simulink library "ad_agg_scalar"  (R2017a)
settings: Solver=VariableStepAuto  StartTime=0.0  StopTime=10.0  RelTol=1e-3
libraries: autodiff x5
settings Model: Creator=eruffaldi  LastModifiedBy=eruffaldi

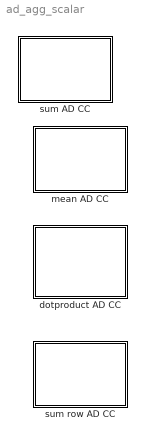
== system ad_agg_scalar ==
  dotproduct AD CC : Subsystem
  mean AD CC : Subsystem
  sum AD CC : Subsystem
  sum row AD CC : Subsystem
      mask Display: disp('Sum by ROW');

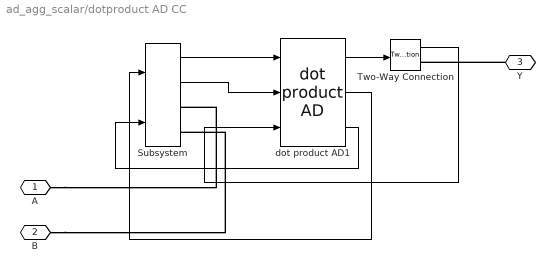
== system ad_agg_scalar/dotproduct AD CC ==
  Subsystem : autodiff/Plus AD CC/Subsystem
      settings: SourceProductName=AutoDiff
  Two-Way Connection : TwoWayConnection
  dot product AD1 : autodiff/dot product AD
      settings: SourceProductName=AutoDiff
  A : PMIOPort  Port=1  Side=Left
  B : PMIOPort  Port=2  Side=Left
  Y : PMIOPort  Port=3  Side=Right
  wires:
  dot product AD1/1 -> Two-Way Connection/1
  dot product AD1/3 -> Subsystem/2
  Subsystem/2 -> dot product AD1/2
  Two-Way Connection/1 -> dot product AD1/3
  dot product AD1/2 -> Subsystem/1
  Subsystem/1 -> dot product AD1/1
  connections:
  Y/RConn1 -- Two-Way Connection/RConn1
  A/RConn1 -- Subsystem/RConn1
  B/RConn1 -- Subsystem/RConn2

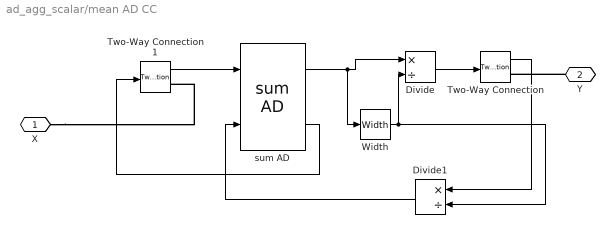
== system ad_agg_scalar/mean AD CC ==
  Divide : Product  Inputs=*/
  Divide1 : Product  Inputs=*/
  Two-Way Connection : TwoWayConnection
  Two-Way Connection1 : TwoWayConnection
  Width : Width
  sum AD : autodiff/sum AD
      settings: SourceProductName=AutoDiff
  X : PMIOPort  Port=1  Side=Left
  Y : PMIOPort  Port=2  Side=Right
  wires:
  sum AD/2 -> Two-Way Connection1/1
  Two-Way Connection1/1 -> sum AD/1
  sum AD/1 -> Width/1, Divide/1
  Divide/1 -> Two-Way Connection/1
  Two-Way Connection/1 -> Divide1/1
  Width/1 -> Divide1/2, Divide/2
  Divide1/1 -> sum AD/2
  connections:
  Y/RConn1 -- Two-Way Connection/RConn1
  X/RConn1 -- Two-Way Connection1/RConn1

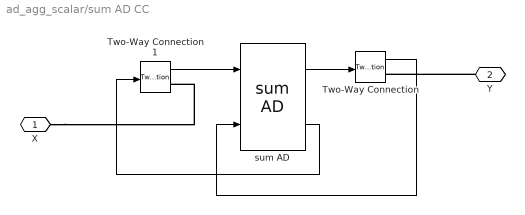
== system ad_agg_scalar/sum AD CC ==
  Two-Way Connection : TwoWayConnection
  Two-Way Connection1 : TwoWayConnection
  sum AD : autodiff/sum AD
      settings: SourceProductName=AutoDiff
  X : PMIOPort  Port=1  Side=Left
  Y : PMIOPort  Port=2  Side=Right
  wires:
  sum AD/1 -> Two-Way Connection/1
  sum AD/2 -> Two-Way Connection1/1
  Two-Way Connection1/1 -> sum AD/1
  Two-Way Connection/1 -> sum AD/2
  connections:
  Y/RConn1 -- Two-Way Connection/RConn1
  X/RConn1 -- Two-Way Connection1/RConn1

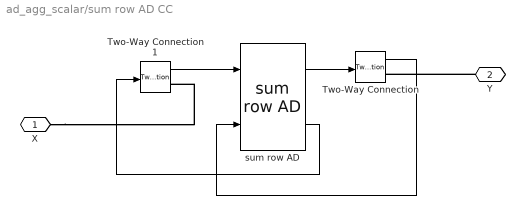
== system ad_agg_scalar/sum row AD CC ==
  Two-Way Connection : TwoWayConnection
  Two-Way Connection1 : TwoWayConnection
  sum row AD : autodiff/sum row AD
      settings: SourceProductName=AutoDiff
  X : PMIOPort  Port=1  Side=Left
  Y : PMIOPort  Port=2  Side=Right
  wires:
  sum row AD/1 -> Two-Way Connection/1
  sum row AD/2 -> Two-Way Connection1/1
  Two-Way Connection1/1 -> sum row AD/1
  Two-Way Connection/1 -> sum row AD/2
  connections:
  Y/RConn1 -- Two-Way Connection/RConn1
  X/RConn1 -- Two-Way Connection1/RConn1
